simulink model "Seminar4_Topic2_3"  (R2019b)
settings: Solver=VariableStepAuto  StartTime=0.0  StopTime=0.05  MaxStep=1e-4  RelTol=1e-3
model workspace (MAT data in the model file):
  d = 16
libraries: powerlib x20
settings Model: Creator=16345  LastModifiedBy=96547
settings DataIOCC: ReturnWorkspaceOutputs=off
settings DebuggingCC: ArithmeticOperatorsInVariantConditions=warning
settings SFSimCC: SimUseLocalCustomCode=off  CustomCodeUndefinedFunction=UseInterfaceOnly
settings RTWCC: RTWUseLocalCustomCode=off

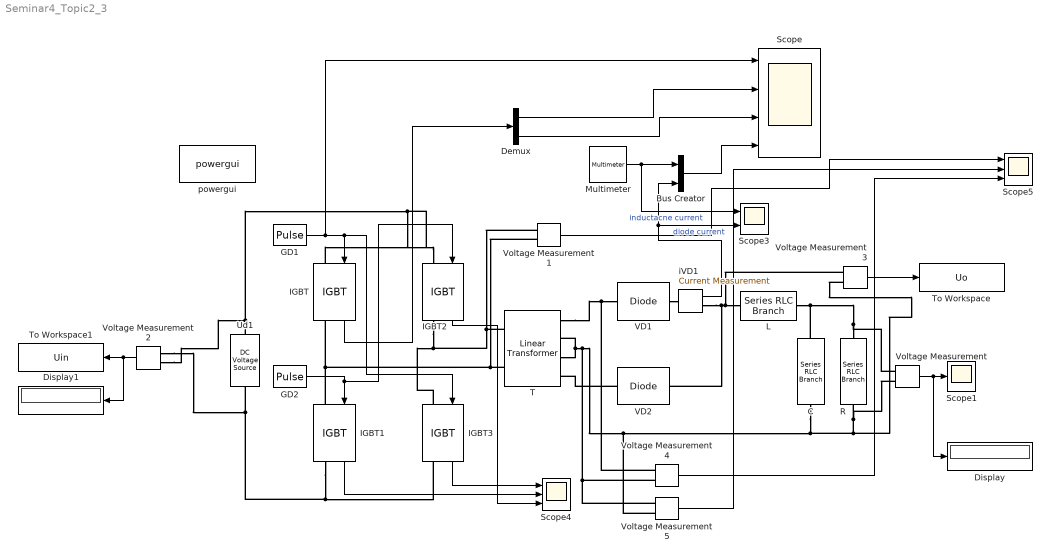
== system Seminar4_Topic2_3 ==
  Bus Creator : BusCreator  DialogController=Simulink.DDGSource_Bus  Inputs=2
  C : powerlib/Elements/Series RLC Branch  LConnTagsString=__new0  RConnTagsString=__new0  BranchType=C  Resistance=0  Inductance=0  SetiL0=off  InitialCurrent=0  Capacitance=2e-4  Setx0=off  InitialVoltage=0  Measurements=None
      settings: SourceProductName=Simscape Electrical
  Demux : Demux  Outputs=2
  Display : Display
  Display1 : Display
  GD1 : DiscretePulseGenerator  PulseType=Time based  Period=1e-5  PulseWidth=16
  GD2 : DiscretePulseGenerator  PulseType=Time based  Period=1e-5  PulseWidth=16  PhaseDelay=5e-6
  IGBT{,1..3} (4 alike) : powerlib/Power Electronics/IGBT  Ron=0  Lon=0  Vf=0  Tf=1e-6  Tt=2e-6  IC=0  Rs=1e5  Cs=inf  Measurements=on
      settings: SourceProductName=Simscape Electrical
  L : powerlib/Elements/Series RLC Branch  LConnTagsString=__new0  RConnTagsString=__new0  BranchType=L  Resistance=0  Inductance=3e-4  SetiL0=off  InitialCurrent=6  Capacitance=inf  Setx0=off  InitialVoltage=0  Measurements=Branch voltage and current
      settings: SourceProductName=Simscape Electrical
  Multimeter : powerlib/Measurements/Multimeter  PhasorSimulation=off  OutputType=Complex  sel=6  L=6  Gain=1  yselected={'Ib: L'};  PSBOutputType=1  PSBequivalent=0  AxesSetting=[0,0.1,-100,100]  Display=0  SavedBlockNames=-11
      settings: SourceProductName=Simscape Electrical
  R : powerlib/Elements/Series RLC Branch  LConnTagsString=__new0  RConnTagsString=__new0  BranchType=R  Resistance=100  Inductance=0  SetiL0=off  InitialCurrent=0  Capacitance=inf  Setx0=off  InitialVoltage=0  Measurements=Branch voltage
      settings: SourceProductName=Simscape Electrical
  Scope : Scope  NumInputPorts=4
  Scope1 : Scope
  Scope3 : Scope  NumInputPorts=2
  Scope4 : Scope  NumInputPorts=3
  Scope5 : Scope  NumInputPorts=3
  T : powerlib/Elements/Linear Transformer  UNITS=pu  NominalPower=[1000 20000 ]  winding1="[ 100  0  0 ]"  winding2="[ 25  0  0 ]"  ThreeWindings=on  winding3=[ 25 0 0 ]  RmLm=[ inf inf ]  Measurements=Winding voltages  DataType=off
      settings: SourceProductName=Simscape Electrical
  To Workspace : ToWorkspace  VariableName=Uo  SampleTime=-1
      settings: Save2DSignal=2-D array (concatenate along first dimension)
  To Workspace1 : ToWorkspace  VariableName=Uin  SampleTime=-1
      settings: Save2DSignal=2-D array (concatenate along first dimension)
  Ud1 : powerlib/Electrical Sources/DC Voltage Source  Amplitude=600  Measurements=None
      settings: SourceProductName=Simscape Electrical
  VD1 : powerlib/Power Electronics/Diode  Ron=0  Lon=0  Vf=0  IC=0  UseSnubber=0  Rs=inf  Cs=1e-9  Measurements=off
      settings: SourceProductName=Simscape Electrical
  VD2 : powerlib/Power Electronics/Diode  Ron=0  Lon=0  Vf=0  IC=0  UseSnubber=0  Rs=inf  Cs=1e-9  Measurements=off
      settings: SourceProductName=Simscape Electrical
  Voltage Measurement{,1..5} (6 alike) : powerlib/Measurements/Voltage Measurement  PhasorSimulation=off  OutputType=Complex  PSBequivalent=0
      settings: SourceProductName=Simscape Electrical
  iVD1 : powerlib/Measurements/Current Measurement  PhasorSimulation=off  OutputType=Complex  PSBequivalent=0
      settings: SourceProductName=Simscape Electrical
  powergui : powerlib/powergui  Priority=1  SimulationMode=Continuous  SampleTime=50e-6  frequency=60  Iterations=50  frequencyindice=0  Pbase=100e6  ErrMax=1e-4  UnitsV=kV  UnitsW=MW  buscounter=0  FunctionMessages=off  echomessages=off  EnableUseOfTLC=off  CurrentSourceSwitches=off  DisableSnubberDevices=off  DisableRonSwitches=off  DisableVfSwitches=off  DisplayEquations=off  AutomaticDiscreteSolvers=off  SolverType=Tustin/Backward Euler (TBE)  Interpol=off  ExternalGateDelay=off  methode=off  Ts=100  x0status=blocks  SPID=on  SwTol=0  HookPort=off  NonlinearTolerance=1e-4  nMaxIteration=100  ContinueOnMaxIteration=off  RestoreLinks=warning  ResistiveCurrentMeasurement=off  Frange=[0:2:500]  Ylog=off  Xlog=on  ShowGrid=off  save=off  variable=ZData  structure=0  ZoomFFT=off  StartTime=0.0  cycles=1  DisplayStyle=1  fundamental=60  FreqAxis=off  MaxFrequency=1000  frequencyindicesteady=1  RmsSteady=1  display=off
      settings: SourceProductName=Simscape Electrical
  wires:
  Multimeter/1 -> Scope3/1, Bus Creator/1  "inductacne current"
  Voltage Measurement/1 -> Display/1, Scope1/1
  Demux/1 -> Scope/2
  iVD1/1 -> Scope3/2, Bus Creator/2  "diode current"
  Bus Creator/1 -> Scope/4
  Demux/2 -> Scope/3
  IGBT/1 -> Demux/1
  GD1/1 -> IGBT3/1, IGBT/1, Scope/1
  GD2/1 -> IGBT2/1, IGBT1/1
  Voltage Measurement1/1 -> Scope5/1
  Voltage Measurement2/1 -> Display1/1, To Workspace1/1
  IGBT3/1 -> Scope4/1
  IGBT1/1 -> Scope4/2
  IGBT2/1 -> Scope4/3
  Voltage Measurement3/1 -> To Workspace/1
  Voltage Measurement4/1 -> Scope5/3
  Voltage Measurement5/1 -> Scope5/2
  connections:
  R/LConn1 -- C/LConn1 -- L/RConn1 -- Voltage Measurement/LConn1
  IGBT2/RConn1 -- IGBT3/LConn1 -- T/LConn1 -- Voltage Measurement1/LConn1
  iVD1/RConn1 -- VD2/RConn1 -- Voltage Measurement3/LConn1 -- L/LConn1
  IGBT/RConn1 -- T/LConn2 -- Voltage Measurement1/LConn2 -- IGBT1/LConn1
  T/RConn2 -- Voltage Measurement5/LConn1 -- Voltage Measurement4/LConn2 -- Voltage Measurement5/LConn2 -- Voltage Measurement3/LConn2 -- Voltage Measurement/LConn2 -- R/RConn1 -- C/RConn1 -- T/RConn3
  IGBT2/LConn1 -- Voltage Measurement2/LConn1 -- Ud1/RConn1 -- IGBT/LConn1
  IGBT1/RConn1 -- Voltage Measurement2/LConn2 -- Ud1/LConn1 -- IGBT3/RConn1
  VD1/RConn1 -- iVD1/LConn1
  VD2/LConn1 -- T/RConn4
  T/RConn1 -- Voltage Measurement4/LConn1 -- VD1/LConn1
